simulink model "Interception_Simulation"  (R2025b)
settings: Solver=FixedStepAuto  StartTime=0.0  StopTime=t_sim  FixedStep=dt_sim  RelTol=1e-3
undefined symbols (not defined in the file or in its folder): dt_sim, t_sim
libraries: simulink_extras x9, MISSILE_GUIDANCE_LIB2 x8, matrix_library x1
settings Model: Creator=leoni  LastModifiedBy=Leonid
settings DataIOCC: SaveFormat=Array
settings RTWCC: GPUComputeCapability=3.5

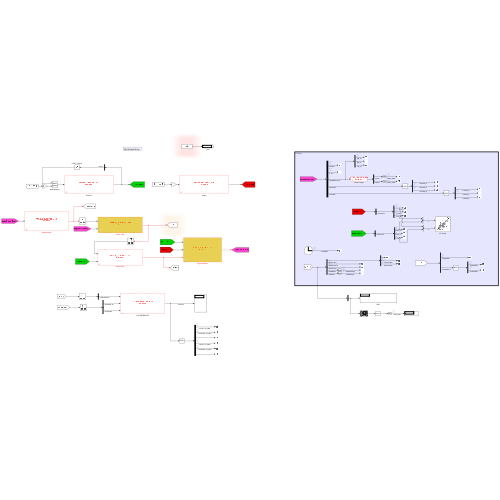
[thumbnail: Simulink's stored preview of the top-level diagram]
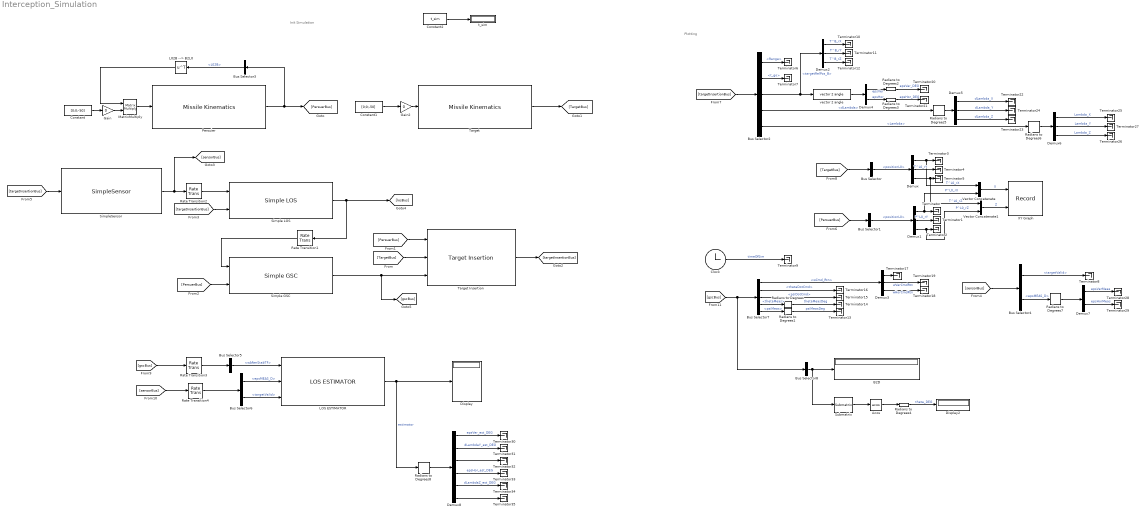
== system Interception_Simulation ==
  note: Plotting
  note: Init Simulation
  Acos : Trigonometry  Operator=acos
  B2D : Display
  Bus Selector : BusSelector  OutputSignals=positionL0
  Bus Selector1 : BusSelector  OutputSignals=positionL0
  Bus Selector2 : BusSelector  OutputSignals=Range,t_go,targetRelPos_B,dLambda,Lambda
  Bus Selector3 : BusSelector  OutputSignals=L02B
  Bus Selector4 : BusSelector  OutputSignals=targetValid,epsMEAS_D
  Bus Selector5 : BusSelector  OutputSignals=wAfterStabTF
  Bus Selector6 : BusSelector  OutputSignals=epsMEAS_D,targetValid
  Bus Selector7 : BusSelector  OutputSignals=wCmd_Rtn,thetaDotCmd,psiDotCmd,thetaMeas,psiMeas
  Bus Selector8 : BusSelector  OutputSignals=B2D  OutputAsBus=on
  Clock : Clock
  Constant : Constant  Value=[0;0;-50]
  Constant1 : Constant  Value=[0;0;-50]
  Constant2 : Constant  Value=t_sim
  Demux{,1..3,5..6} (6 alike) : Demux  Outputs=3
  Demux4 : Demux  Outputs=2
  Demux7 : Demux  Outputs=2
  Demux8 : Demux  Outputs=6
  Display : Display
  Display2 : Display
  Gain : Gain  Gain=0
  Gain2 : Gain  Gain=0
  L02B --> B2L0 : Math  Operator=transpose
  LOS ESTIMATOR : MISSILE_GUIDANCE_LIB2/LOS ESTIMATOR  Q=100  R=0.1
  MatrixMultiply : Product  Multiplication=Matrix(*)
  Persuier : MISSILE_GUIDANCE_LIB2/Missile Kinematics  psi0_theta0_phi0=[0;0;0]  vX0=0  r0=[0;0;0]  tau_X=0.1  tau_YZ=0.1
  Radians to Degrees{,1..8} (9 alike) : simulink_extras/Transformations/Radians to Degrees
  Rate Transition{1..4} (4 alike) : RateTransition
  Simple GSC : MISSILE_GUIDANCE_LIB2/Simple GSC  theta0=5  psi0=0  fRATE=25  zetaRATE=0.7  f_clock_GSC=1800  enErrors=off  errorsVec=(rand(9,1)*2-1)*25*1e-3  Jo_kgmm=4000  Ji_kgmm=3000  Icmd_MAX=4.0  Kt_mNm=50
  Simple LOS : MISSILE_GUIDANCE_LIB2/Simple LOS  kLOS=5  f_clock_LOS=600  perfectPoint=on  perfectTrack=on
  SimpleSensor : MISSILE_GUIDANCE_LIB2/SimpleSensor  halfFov=4  epsNoise=0  rangeNoise=0  rangeDotNoise=0  f_clock_SENS=100  tLatency=dt_sim*1000
  Submatrix : matrix_library/Submatrix  RowSpan=One row  RowStartMode=Last  RowStartIndex=1  RowEndMode=Last  RowEndIndex=1  ColSpan=One column  ColStartMode=Last  ColStartIndex=1  ColEndMode=Last  ColEndIndex=1
  Target : MISSILE_GUIDANCE_LIB2/Missile Kinematics  psi0_theta0_phi0=[0;0;0]  vX0=0  r0=[1000;0;-364]  tau_X=1  tau_YZ=1
  Target Insertion : MISSILE_GUIDANCE_LIB2/Target Insertion
  Terminator{,1..35} (36 alike) : Terminator
  Vector Concatenate : Concatenate
  Vector Concatenate1 : Concatenate
  XY Graph : Record  NumPorts=2.0  FileSettingsInternal="{\"entries\":[{\"content\":{\"excelSettings\":{\"content\":{},\"type\":\"Streamout.ExcelSettings\"},\"parquetSettings\":{\"content\":{},\"type\":\"Streamout.ParquetSettings\"}},\"type\":\"Streamout.FileSettingStorage\",\"uuid\":\"\"}],\"packageUris\":[\"http:\\/\\/schema.mathworks.com\\/mf0\\/streamout_blocks\\/R2020a\"],\"version\":\"1.0\"}"  FrameSettings=[0, 0]  Layout=[1 1]  SignalsInternal="{\"entries\":[{\"content\":{\"signals\":[{\"content\":{\"blockPath\":[],\"dimensions\":[2],\"domain\":\"\",\"hasChildren\":true,\"lineColor\":\"#22b573\",\"lineWidth\":2,\"port\":1,\"signalID\":1,\"signalName\":\"X\"},\"type\":\"RecordBlkView.Signal\",\"uuid\":\"\"},{\"content\":{\"blockPath\":[],\"channel\":[1],\"dimensions\":[2],\"domain\":\"\",\"lineColor\":\"#fe330a\",\"parentID\":1,\"plots\":[ 1 ],\"port\":1,\"signalID\":2,\"signalName\":\"X\"},\"type\":\"RecordBlkView.Signal\",\"uuid\":\"\"},{\"content\":{\"blockPath\":[],\"channel\":[2],\"dimensions\":[2],\"domain\":\"\",\"lineColor\":\"#22b573\",\"parentID\":1,\"plots\":[ 1 ],\"port\":1,\"signalID\":3,\"signalName\":\"X\"},\"type\":\"RecordBlkView.Signal\",\"uuid\":\"\"},{\"content\":{\"blockPath\":[],\"dimensions\":[2],\"domain\":\"\",\"hasChildren\":true,\"lineColor\":\"#d95319\",\"lineWidth\":2,\"port\":2,\"signalID\":4,\"signalName\":\"Z\"},\"type\":\"RecordBlkView.Signal\",\"uuid\":\"\"},{\"content\":{\"blockPath\":[],\"channel\":[1],\"dimensions\":[2],\"domain\":\"\",\"lineColor\":\"#fe330a\",\"parentID\":4,\"plots\":[ 1 ],\"port\":2,\"signalID\":5,\"signalName\":\"Z\"},\"type\":\"RecordBlkView.Signal\",\"uuid\":\"\"},{\"content\":{\"blockPath\":[],\"channel\":[2],\"dimensions\":[2],\"domain\":\"\",\"lineColor\":\"#22b573\",\"parentID\":4,\"plots\":[ 1 ],\"port\":2,\"signalID\":6,\"signalName\":\"Z\"},\"type\":\"RecordBlkView.Signal\",\"uuid\":\"\"}]},\"type\":\"RecordBlkView.InputSignals\",\"uuid\":\"\"}],\"packageUris\":[\"http:\\/\\/schema.mathworks.com\\/mf0\\/streamout_blocks\\/R2020a\"],\"version\":\"1.0\"}"  VisualizationBindings="{\"xyplotplugin\":{\"info\":[{\"series\":[{\"bindingParametersList\":[{\"parameter\":\"X-Axis\",\"signalID\":2,\"signalName\":\"X(1)\"},{\"parameter\":\"Y-Axis\",\"signalID\":5,\"signalName\":\"Z(1)\"}],\"seriesID\":0},{\"bindingParametersList\":[{\"parameter\":\"X-Axis\",\"signalID\":3,\"signalName\":\"X(2)\"},{\"parameter\":\"Y-Axis\",\"signalID\":6,\"signalName\":\"Z(2)\"}],\"seriesID\":1}],\"subplotID\":1}]}}"  CompatibilityTag=XY
  t_sim : Display
  vector 2 angle : MISSILE_GUIDANCE_LIB2/vector 2 angle  SystemSampleTime=-1  VariantActivationTime=update diagram  EmptyChoice=off  PassThrough=off  PassThroughVariantControl=(default)  EmptyChoiceVariantControl=(default)  AllowFlexibleInterface=on  Latency=0  AutoFrameSizeCalculation=off
  wires:
  Bus Selector/1 -> Demux/1  "<positionL0>"
  Demux/1 -> Vector Concatenate/1, Terminator3/1  "T^L0_rX"
  Demux/2 -> Terminator4/1  "T^L0_rY"
  Demux/3 -> Vector Concatenate1/1, Terminator5/1  "T^L0_rZ"
  Bus Selector1/1 -> Demux1/1  "<positionL0>"
  Demux1/1 -> Vector Concatenate/2, Terminator/1  "P^L0_rX"
  Demux1/2 -> Terminator1/1  "P^L0_rY"
  Demux1/3 -> Vector Concatenate1/2, Terminator2/1  "P^L0_rZ"
  Bus Selector2/1 -> Terminator6/1  "<Range>"
  Bus Selector2/2 -> Terminator7/1  "<t_go>"
  Constant/1 -> Gain/1
  Constant1/1 -> Gain2/1
  Bus Selector3/1 -> L02B --> B2L0/1  "<L02B>"
  L02B --> B2L0/1 -> MatrixMultiply/1
  Persuier/1 -> Bus Selector3/1, [PersuerBus]
  Target/1 -> [TargetBus]
  [TargetBus] -> Target Insertion/2
  [PersuerBus] -> Target Insertion/1
  Target Insertion/1 -> [targetInsertionBus]
  [PersuerBus] -> Simple GSC/2
  Simple LOS/1 -> [losBus], Rate Transition1/1
  [targetInsertionBus] -> Simple LOS/2
  [targetInsertionBus] -> SimpleSensor/1
  [PersuerBus] -> Bus Selector1/1
  [targetInsertionBus] -> Bus Selector2/1
  [TargetBus] -> Bus Selector/1
  MatrixMultiply/1 -> Persuier/1
  SimpleSensor/1 -> [sensorBus], Rate Transition2/1
  Simple GSC/1 -> [gscBus], Target Insertion/3
  Rate Transition1/1 -> Simple GSC/1
  Rate Transition2/1 -> Simple LOS/1
  [sensorBus] -> Bus Selector4/1
  Bus Selector4/1 -> Terminator8/1  "<targetValid>"
  Clock/1 -> Terminator9/1  "timeOfSim"
  [gscBus] -> Rate Transition3/1
  Bus Selector5/1 -> LOS ESTIMATOR/1  "<wAfterStabTF>"
  [sensorBus] -> Rate Transition4/1
  Bus Selector6/1 -> LOS ESTIMATOR/2  "<epsMEAS_D>"
  Bus Selector6/2 -> LOS ESTIMATOR/3  "<targetValid>"
  Rate Transition3/1 -> Bus Selector5/1
  Rate Transition4/1 -> Bus Selector6/1
  LOS ESTIMATOR/1 -> Radians to Degrees8/1, Display/1  "estimator"
  Gain/1 -> MatrixMultiply/2
  Gain2/1 -> Target/1
  Bus Selector2/3 -> Demux2/1, vector 2 angle/1  "<targetRelPos_B>"
  Demux2/2 -> Terminator11/1  "T^B_rY"
  Demux2/3 -> Terminator12/1  "T^B_rZ"
  Demux2/1 -> Terminator10/1  "T^B_rX"
  [gscBus] -> Bus Selector8/1, Bus Selector7/1
  Bus Selector7/1 -> Demux3/1  "<wCmd_Rtn>"
  Bus Selector7/2 -> Terminator16/1  "<thetaDotCmd>"
  Bus Selector7/3 -> Terminator15/1  "<psiDotCmd>"
  Bus Selector7/4 -> Radians to Degrees/1  "<thetaMeas>"
  Bus Selector7/5 -> Radians to Degrees1/1  "<psiMeas>"
  Demux3/1 -> Terminator17/1
  Demux3/2 -> Terminator19/1  "wVerCmdRtn"
  Demux3/3 -> Terminator18/1  "wHorCmdRtn"
  Radians to Degrees/1 -> Terminator14/1  "thetaMeasDeg"
  Radians to Degrees1/1 -> Terminator13/1  "psiMeasDeg"
  vector 2 angle/1 -> Demux4/1
  Demux4/1 -> Radians to Degrees2/1  "epsVer"
  Demux4/2 -> Radians to Degrees3/1  "epsHor"
  Radians to Degrees2/1 -> Terminator20/1  "epsVer_DEG"
  Radians to Degrees3/1 -> Terminator21/1  "epsHor_DEG"
  Bus Selector8/1 -> Submatrix/1, B2D/1
  Submatrix/1 -> Acos/1
  Acos/1 -> Radians to Degrees4/1
  Radians to Degrees4/1 -> Display2/1  "theta_DEG"
  Constant2/1 -> t_sim/1
  Vector Concatenate/1 -> XY Graph/1  "X"
  Vector Concatenate1/1 -> XY Graph/2  "Z"
  Bus Selector2/4 -> Radians to Degrees5/1  "<dLambda>"
  Demux5/1 -> Terminator22/1  "dLambda_X"
  Demux5/2 -> Terminator24/1  "dLambda_Y"
  Demux5/3 -> Terminator23/1  "dLambda_Z"
  Radians to Degrees5/1 -> Demux5/1
  Bus Selector2/5 -> Radians to Degrees6/1  "<Lambda>"
  Demux6/3 -> Terminator26/1  "Lambda_Z"
  Demux6/2 -> Terminator27/1  "Lambda_Y"
  Demux6/1 -> Terminator25/1  "Lambda_X"
  Radians to Degrees6/1 -> Demux6/1
  Bus Selector4/2 -> Radians to Degrees7/1  "<epsMEAS_D>"
  Demux7/1 -> Terminator28/1  "epsVerMeas"
  Demux7/2 -> Terminator29/1  "epsHorMeas"
  Radians to Degrees7/1 -> Demux7/1
  Demux8/2 -> Terminator31/1  "dLambdaY_est_DEG"
  Demux8/3 -> Terminator32/1
  Demux8/4 -> Terminator33/1  "epsHor_est_DEG"
  Demux8/5 -> Terminator34/1  "dLambdaZ_est_DEG"
  Demux8/6 -> Terminator35/1
  Demux8/1 -> Terminator30/1  "epsVer_est_DEG"
  Radians to Degrees8/1 -> Demux8/1
